simulink model "X"  (R2016a)
settings: Solver=VariableStepAuto  StartTime=0.0  StopTime=1000  RelTol=1e-3
libraries: simCryogenics_lib x6, nesl_utility x4
settings Model: Creator=FB229602  LastModifiedBy=FB229602
settings GRTTargetCC: GeneratePreprocessorConditionals=Use local settings
settings SimscapeCC: SimscapeLogType=all  SimscapeLogOpenViewer=on  SimscapeLogLimitData=off

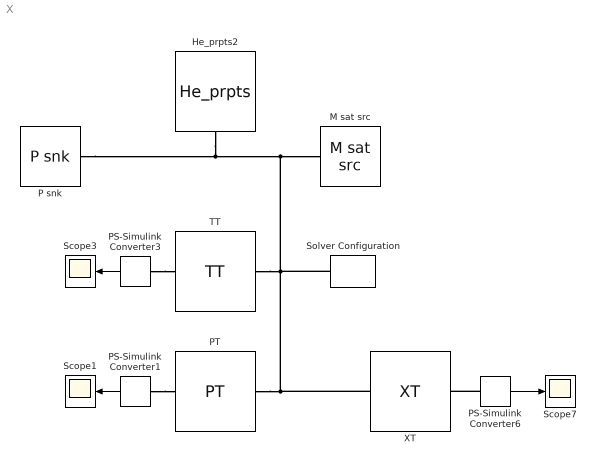
== system X ==
  He_prpts2 : simCryogenics_lib/Utilities/He_prpts  P_min=0.2 bar  T_min=1 K  T_max=100 K  P_max=50 bar  Mol=4.0026 * (10 ^ (- 3)) kg/mol
  M sat src : simCryogenics_lib/Sources_Sinks/M sat src  M=0.1 kg/s  Xmix=0.2
  P snk : simCryogenics_lib/Sources_Sinks/P snk  P=1.5 bar
  PS-Simulink Converter1 : nesl_utility/PS-Simulink Converter  PhysicalDomain=network_engine_domain  SubClassName=ps_output  LeftPortType=input  RightPortType=output  PseudoPeriodic=off  Frequencies=[]  Unit=1  AffineConversion=off
  PS-Simulink Converter3 : nesl_utility/PS-Simulink Converter  PhysicalDomain=network_engine_domain  SubClassName=ps_output  LeftPortType=input  RightPortType=output  PseudoPeriodic=off  Frequencies=[]  Unit=1  AffineConversion=off
  PS-Simulink Converter6 : nesl_utility/PS-Simulink Converter  PhysicalDomain=network_engine_domain  SubClassName=ps_output  LeftPortType=input  RightPortType=output  PseudoPeriodic=off  Frequencies=[]  Unit=1  AffineConversion=off
  PT : simCryogenics_lib/Sensors/PT
  Scope1 : Scope
  Scope3 : Scope
  Scope7 : Scope
  Solver Configuration : nesl_utility/Solver Configuration  PhysicalDomain=network_engine_domain  SubClassName=solver  LeftPortType=input  RightPortType=generic  Accelerate=off  Tones=[]  Harmonics=[]  SimulateNoise=off  Profile=off  UseLocalSampling=off  EnableSwitchedLinearOptims=on  FrequencyDomain=off  UseCCode=off  RelTol=0.001  AbsTol=1e-06  MinStep=1e-09  ToWorkspace=off  RevertToSquareIcSolve=off  NumHomotopyIterations=100  PhasorMode=off  PhasorModeNumHarmonics=1  OverrideAbsTol=off  DoDC=off  ResidualTolerance=1e-09  UseLocalSolver=off  LocalSolverChoice=NE_BACKWARD_EULER_ADVANCER  LocalSolverSampleTime=0.001  DoFixedCost=off  MaxNonlinIter=3  MaxModeIter=2  LinearAlgebra=Sparse  DelaysMemoryBudget=1024  AutomaticFiltering=on  FilteringTimeConstant=0.001
  TT : simCryogenics_lib/Sensors/TT
  XT : simCryogenics_lib/Sensors/XT
  wires:
  PS-Simulink Converter3/1 -> Scope3/1
  PS-Simulink Converter6/1 -> Scope7/1
  PS-Simulink Converter1/1 -> Scope1/1
  connections:
  PS-Simulink Converter3/LConn1 -- TT/RConn1
  PS-Simulink Converter6/LConn1 -- XT/RConn1
  P snk/RConn1 -- Solver Configuration/RConn1 -- TT/LConn1 -- PT/LConn1 -- XT/LConn1 -- M sat src/RConn1 -- He_prpts2/RConn1
  PS-Simulink Converter1/LConn1 -- PT/RConn1
